simulink model "Simulink_Regu"  (R2019b)
settings: Solver=VariableStepAuto  StartTime=0.0  StopTime=10.0  RelTol=1e-3
undefined symbols (not defined in the file): A, Ke, Ks
settings Model: Creator=serbogr1  LastModifiedBy=serbogr1

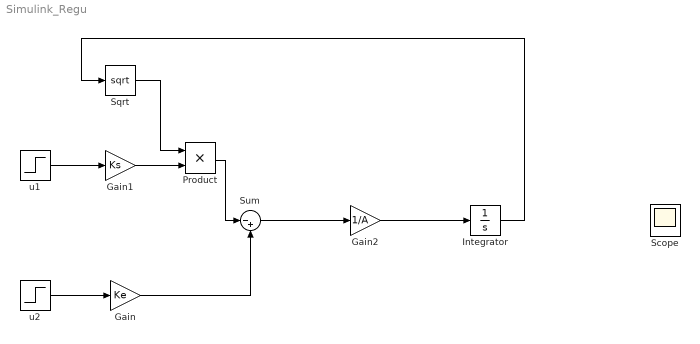
== system Simulink_Regu ==
  Gain : Gain  Gain=Ke
  Gain1 : Gain  Gain=Ks
  Gain2 : Gain  Gain=1/A
  Integrator : Integrator
  Product : Product
  Scope : Scope
  Sqrt : Sqrt  SaturateOnIntegerOverflow=on
  Sum : Sum  Inputs=|-+
  "u1 " : Step  SampleTime=0
  "u2 " : Step  SampleTime=0
  wires:
  Gain/1 -> Sum/2
  "u2 "/1 -> Gain/1
  "u1 "/1 -> Gain1/1
  Gain1/1 -> Product/2
  Sqrt/1 -> Product/1
  Integrator/1 -> Sqrt/1
  Sum/1 -> Gain2/1
  Gain2/1 -> Integrator/1
  Product/1 -> Sum/1
